simulink model "stanleySimple"  (R2022b)
settings: Solver=VariableStepAuto  StartTime=0.0  StopTime=inf  FixedStep=0.001  RelTol=1e-3
PreLoadFcn:
  | setUpModel
  | close
model workspace (MAT data in the model file):
  firstWarning = 0
  originalScenarioChecksum = 'F73A6DA3C723D3CA73A6F931B7A52A9C'
undefined symbols (not defined in the file or in its folder): Angular, esc, hz, K, Linear, path, Ve, Vx
libraries: robotlib x4, dspstat3 x1
settings Model: Creator=valakshe  LastModifiedBy=kishor
settings SolverCC: AlgebraicLoopSolver=TrustRegion
settings DebuggingCC: UnconnectedInputMsg=warning  UnconnectedOutputMsg=warning  UnconnectedLineMsg=warning  SFMachineParentedDataDiag=warning
settings ModelReferenceCC: EnableRefExpFcnMdlSchedulingChecks=on
settings RTWCC: DLArmComputeVersion=19.05

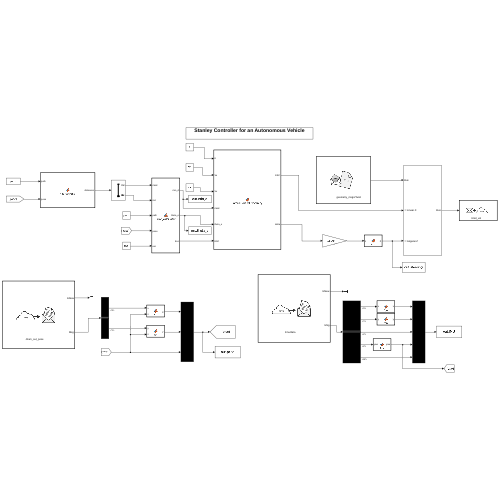
[thumbnail: Simulink's stored preview of the top-level diagram]
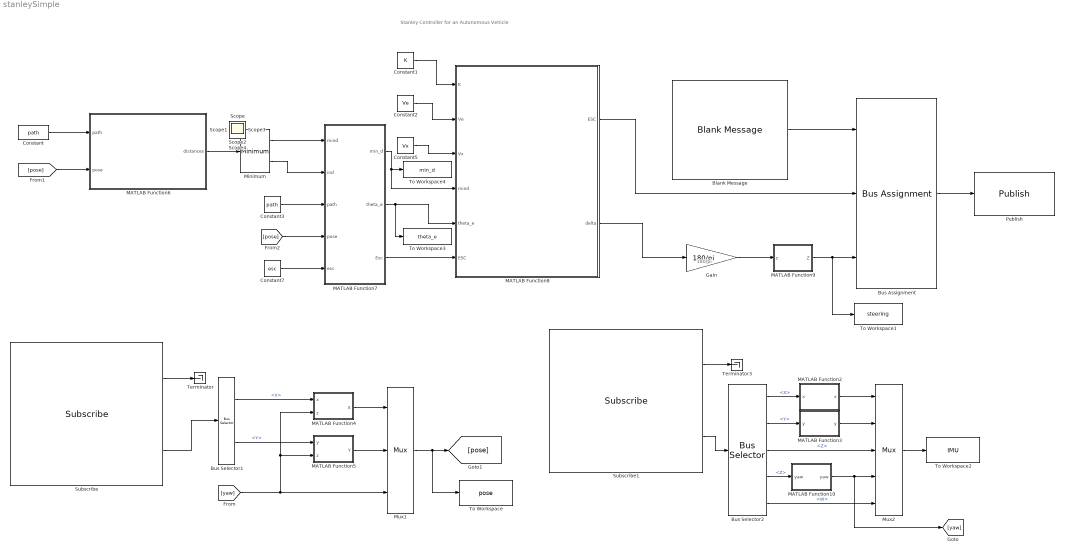
== system stanleySimple ==
  note: 180/pi
  note: Stanley Controller for an Autonomous Vehicle
  Blank Message : robotlib/Blank Message  messageClass=Message  entityType=geometry_msgs/Twist  messageType=geometry_msgs/Twist  SampleTime=1/hz  legacyBusStruct=off
      settings: LibrarySourceBlock=roslib/ROS/Blank Message
  Bus Assignment : BusAssignment  AssignedSignals=Linear.X,Angular.Z
  Bus Selector1 : BusSelector  OutputSignals=Pose.Position.X,Pose.Position.Y
  Bus Selector2 : BusSelector  OutputSignals=LinearAcceleration.X,LinearAcceleration.Y,AngularVelocity.Z,Orientation.Z,Orientation.W
  Constant : Constant  Value=path  SampleTime=1/hz
  Constant1 : Constant  Value=K  SampleTime=1/hz
  Constant2 : Constant  Value=Ve  SampleTime=1/hz
  Constant3 : Constant  Value=path  SampleTime=1/hz
  Constant5 : Constant  Value=Vx  SampleTime=1/hz
  Constant7 : Constant  Value=esc  SampleTime=1/hz
  Gain : Gain  Gain=180/pi
  MATLAB Function10 : MATLAB Function  TreatAsAtomicUnit=on
  MATLAB Function2 : MATLAB Function  TreatAsAtomicUnit=on
  MATLAB Function3 : MATLAB Function  TreatAsAtomicUnit=on
  MATLAB Function4 : MATLAB Function  TreatAsAtomicUnit=on
  MATLAB Function5 : MATLAB Function  TreatAsAtomicUnit=on
  MATLAB Function6 : MATLAB Function  TreatAsAtomicUnit=on
  MATLAB Function7 : MATLAB Function  TreatAsAtomicUnit=on
  MATLAB Function8 : MATLAB Function  TreatAsAtomicUnit=on
  MATLAB Function9 : MATLAB Function  TreatAsAtomicUnit=on
  Minimum : dspstat3/Minimum  operation=minimum  fcn=Value and Index  indexBase=One  operateOver=Each row  Dimension=1  InputProcessing=Columns as channels (frame based)  reset=None  roiEnable=off  roiType=Rectangles  roiPortion=Entire ROI  roiOutput=Individual statistics for each ROI  roiFlag=off  roundingMode=Floor  overflowMode=off
  Mux1 : Mux  Inputs=3
  Mux2 : Mux  Inputs=5
  Publish : robotlib/Publish  topicSource=Specify your own  topic=/cmd_vel  messageType=geometry_msgs/Twist  legacyBusStruct=off  messageQueueLength=1
      settings: LibrarySourceBlock=roslib/ROS/Publish
  Subscribe : robotlib/Subscribe  topicSource=Specify your own  topic=/slam_out_pose  messageType=geometry_msgs/PoseStamped  SampleTime=1/hz  legacyBusStruct=off  messageQueueLength=1
      settings: LibrarySourceBlock=roslib/ROS/Subscribe
  Subscribe1 : robotlib/Subscribe  topicSource=Specify your own  topic=/imu/data  messageType=sensor_msgs/Imu  SampleTime=1/hz  legacyBusStruct=off  messageQueueLength=1
      settings: LibrarySourceBlock=roslib/ROS/Subscribe
  Terminator : Terminator
  Terminator3 : Terminator
  To Workspace : ToWorkspace  VariableName=pose  SaveFormat=Structure With Time  SampleTime=-1
  To Workspace1 : ToWorkspace  VariableName=steering  SaveFormat=Structure With Time  SampleTime=1/hz
  To Workspace2 : ToWorkspace  VariableName=IMU  SaveFormat=Structure With Time  SampleTime=-1
  To Workspace3 : ToWorkspace  VariableName=theta_e  SaveFormat=Structure With Time  SampleTime=-1
  To Workspace4 : ToWorkspace  VariableName=min_d  SaveFormat=Structure With Time  SampleTime=-1
  Scope{,1..4} (5 alike) : Scope
  wires:
  Bus Assignment/1 -> Publish/1
  Blank Message/1 -> Bus Assignment/1
  Gain/1 -> MATLAB Function9/1(z)
  [pose] -> MATLAB Function6/2(pose)
  Constant/1 -> MATLAB Function6/1(path)
  MATLAB Function6/1(distances) -> Minimum/1
  Minimum/1 -> MATLAB Function7/1(mind)
  Minimum/2 -> MATLAB Function7/2(ind)
  Constant3/1 -> MATLAB Function7/3(path)
  [pose] -> MATLAB Function7/4(pose)
  MATLAB Function7/2(theta_e) -> To Workspace3/1, MATLAB Function8/5(theta_e)
  MATLAB Function7/1(min_d) -> To Workspace4/1, MATLAB Function8/4(mind)
  Constant1/1 -> MATLAB Function8/1(K)
  Constant2/1 -> MATLAB Function8/2(Ve)
  Constant5/1 -> MATLAB Function8/3(Vx)
  MATLAB Function7/3(Esc) -> MATLAB Function8/6("ESC ")
  Constant7/1 -> MATLAB Function7/5(esc)
  MATLAB Function8/2(delta) -> Gain/1
  MATLAB Function8/1(ESC) -> Bus Assignment/2
  MATLAB Function9/1(Z) -> To Workspace1/1, Bus Assignment/3
  Subscribe/1 -> Terminator/1
  Bus Selector2/4 -> MATLAB Function10/1("yaw ")  "<Z>"
  Bus Selector1/1 -> MATLAB Function4/1(x)  "<X>"
  MATLAB Function10/1(yaw) -> Mux2/4, [yaw]
  MATLAB Function4/1(X) -> Mux1/1
  MATLAB Function3/1(y) -> Mux2/2
  Bus Selector2/1 -> MATLAB Function2/1("x ")  "<X>"
  Bus Selector2/2 -> MATLAB Function3/1("y ")  "<Y>"
  Subscribe1/1 -> Terminator3/1
  Subscribe/2 -> Bus Selector1/1
  Bus Selector1/2 -> MATLAB Function5/1(y)  "<Y>"
  Mux1/1 -> To Workspace/1, [pose]
  [yaw] -> Mux1/3, MATLAB Function5/2(z), MATLAB Function4/2(z)
  MATLAB Function5/1(Y) -> Mux1/2
  MATLAB Function2/1(x) -> Mux2/1
  Mux2/1 -> To Workspace2/1
  Subscribe1/2 -> Bus Selector2/1
  Bus Selector2/5 -> Mux2/5  "<W>"
  Bus Selector2/3 -> Mux2/3  "<Z>"

== matlab function stanleySimple/MATLAB Function10 ==
  data: yaw input; yaw output
function yaw = fcn(yaw)
yaw = 360-yaw;
yaw = yaw*pi/180;
end

== matlab function stanleySimple/MATLAB Function2 ==
  data: x input; x output
function x = fcn(x)
x = x - (0);
end

== matlab function stanleySimple/MATLAB Function4 ==
  data: x input; X output; z input
function X = fcn(x,z)

X = x + 0.325*cos(z);

end

== matlab function stanleySimple/MATLAB Function5 ==
  data: y input; Y output; z input
function Y = fcn(y,z)
Y = y + 0.325*sin(z);
end

== matlab function stanleySimple/MATLAB Function6 ==
  data: path input; distances output; pose input
function distances  = nearestPose(path, pose)
    % path: Nx3 matrix containing the x, y, and heading of the waypoints in the path
    % current_pose: 1x3 vector containing the x, y, and heading of the current pose of the vehicle
    % nearest_pose: 1x3 vector containing the x, y, and heading of the nearest pose on the path
    % nearest_index: index of the nearest pose on the path
    
    % Find the distance from the current pose to each waypoint on the path
    
    l = length(path(:,1));
    cx = path(:,1);
    cy = path(:,2);
    dx = zeros(1,l);
    dy = zeros(1,l);
    distances =  zeros(1,l);


    for i = 1:l
        dx(i) = pose(1) - cx(i);
        dy(i) = pose(2) - cy(i);
        distances(i) = sqrt((dx(i)^2+dy(i)^2));
    end
end

== matlab function stanleySimple/MATLAB Function7 ==
  data: mind input; ind input; min_d output; path input; pose input; theta_e output; esc input; Esc output
function [min_d,theta_e,Esc]  = Error_calculator(mind,ind,path,pose,esc)
%%%%%%%%%%%%%%%%%%%%%%%%%%%%%%%%%%%%%%%%%%%%%%%%%%%%%%%%%%%
theta_pose = pose(3);
theta_ref = path(ind,3);
theta_e = theta_ref - theta_pose;
if theta_e <= -pi
    theta_e = theta_ref + (2*pi-theta_pose); 
elseif theta_e >= pi
    theta_e = -(2*pi-theta_ref + theta_pose);

end


%%%%%%%%%%%%%%%%%%%%%%%%%%%%%%%%%%%%%%%%%%%%%%%%%%%%%%%%%%%%

current_position = [pose(1);pose(2)];
next_waypoint = [path(ind+1,1);path(ind+1,2)];

waypoint_vector = next_waypoint - current_position;
normal_vector = [-waypoint_vector(2), waypoint_vector(1)];
vehicle_heading = [cos(pose(3)), sin(pose(3))];
dot_product = dot(vehicle_heading, normal_vector);
if dot_product > 0
    cross_track_error = -1; % vehicle is to the right of the line
else
    cross_track_error = +1; % vehicle is to the left of the line
end
min_d = mind*cross_track_error;

%%%%%%%%%%%%%%%%%%%%%%%%%%%%%%%%%
if ind >= length(path(:,1))-20
    Esc = 0;
    min_d = 0;
    theta_e = 0;
    path(ind+5,1)
    
else
    Esc = esc;
end

== matlab function stanleySimple/MATLAB Function8 ==
  data: ESC output; K input; Ve input; Vx input; mind input; theta_e input; delta output; ESC input
function [ESC,delta] = LateralControllerStanley(K,Ve,Vx,mind,theta_e,ESC)

delta = theta_e + atan(K*mind/(Ve+Vx));
%b = atan(K*mind/(Ve+Vx))*180/pi
%a = theta_e*180/pi
end

== matlab function stanleySimple/MATLAB Function9 ==
  data: z input; Z output
function Z = fcn(z)

if (z > 30)
    z = 30;
elseif (z < -30)
    z = -30;
else
    z =z;
end

Z = z;
end

== matlab function stanleySimple/MATLAB Function3 ==
  data: y input; y output
function y = fcn(y)
y = y - (0);
end
